simulink library "SUB_ECU_L4_MABX_HW_Interface"  (R2018a)
settings: Solver=VariableStepAuto  StartTime=0.0  StopTime=10.0  RelTol=1e-3
PostLoadFcn:
  | , if any(exist('dsrtsu_mdlpostloadfcn', 'file') == [2, 3, 6]), try dsrtsu_mdlpostloadfcn('Execute', bdroot); catch fprintf('Error in PostLoadFcn (dsrtsu_mdlpostloadfcn) for model "%s":\n %s\n', bdroot, lasterr); end, end,
undefined symbols (not defined in the file or in its folder): CANR_PROPB_REAX_3_13_CHANNEL_APV, CANR_PROPB_REAX_4_13_CHANNEL_APV, CANR_PROPB_XPR_1_50_CHANNEL_APV, ENUM_CAN_RX_T, ENUM_CAN_TX_T, ENUM_REAX_OPERATION_MODE_T, ENUM_SIGNAL_HEALTH_T, ENUM_XBR_CONTROL_MODE_T, ENUM_XBR_EBI_MODE_T, ENUM_XBR_PASS_THROUGH_ACTIVE_T, ENUM_XBR_PRIORITY_T, ENUM_XPR_INHIBIT_PARK_MANUAL_T, ENUM_XPR_INHIBIT_UNPARK_MANUAL_T, ENUM_XPR_PARK_MANUAL_T, ENUM_XPR_UNPARK_MANUAL_T, PROPB_REAX_1_E4_DES_POS_SIG_SRC_APV, PROPB_REAX_1_E4_DESIRED_OPMODE_APV, PROPB_REAX_1_E4_DESIRED_POSITION_APV, ptc_matlab_lib
libraries: PTC_MBDS_LIB x264, rtican x172, EmE_MBD_Blockset x39, simulink x34, $bdroot x16, rti1401lib_dio_type4 x8, simulink_need_slupdate x7, dsa_tcpip_lib x4, rti1401lib_adc_type4 x3, rtmapslib x3, rtitasklib x3
(part 9 of 51)

== system SUB_ECU_L4_MABX_HW_Interface/CAN_Out_PTC_1571/CAN_TX_10ms/Encode_PROPB_REAX_1 ==
  In1 : Inport
  Bus Selector : BusSelector  OutputSignals=10msTask.SteeringControl.DesSteeringAngle
  Bus Selector1 : BusSelector  OutputSignals=INPUTS.DIO_Bus.OperatorEnableSwitch
  CAN_ID_PropB_REAX_1_E4 : Subsystem
  Data Type Conversion : DataTypeConversion  OutDataTypeStr=uint8
  Encode_PROPB_REAX_1 : Subsystem
  PropB_REAX_1_E4_CommandFromExternalController : Subsystem
  PropB_REAX_1_E4_DesiredOperatingMode : Subsystem
  PropB_REAX_1_E4_MessageCounter : Subsystem
  Out1 : Outport
  wires:
  Data Type Conversion/1 -> PropB_REAX_1_E4_CommandFromExternalController/2(operatorEnable), PropB_REAX_1_E4_DesiredOperatingMode/1(OperatorEnable)
  Bus Selector/1 -> PropB_REAX_1_E4_CommandFromExternalController/1(DesiredSteeringAngle)  "<DesSteeringAngle>"
  Bus Selector1/1 -> Data Type Conversion/1  "<OperatorEnableSwitch>"
  CAN_ID_PropB_REAX_1_E4/1(MessageID) -> Encode_PROPB_REAX_1/1(MessageID)
  PropB_REAX_1_E4_DesiredOperatingMode/1(DesiredOperatingMode) -> Encode_PROPB_REAX_1/2(DesiredOperatingMode)
  Encode_PROPB_REAX_1/1(Data) -> Out1/1
  PropB_REAX_1_E4_MessageCounter/1(MessageCounter) -> Encode_PROPB_REAX_1/4(MessageCounter)
  PropB_REAX_1_E4_CommandFromExternalController/1(CommandFromExternalController) -> Encode_PROPB_REAX_1/3(CommandFromExternalController)
  In1/1 -> Bus Selector1/1, Bus Selector/1

== system SUB_ECU_L4_MABX_HW_Interface/CAN_Out_PTC_1571/CAN_TX_20ms/CAN_TX_PROPB_XBR_B3 ==
  Channel : Inport
  Data : Inport  Port=2
  OperatorEnable : Inport  Port=3
  AND : PTC_MBDS_LIB/MBDS Standard Library/Basic Operations/Logic and Bit Operations/AND  BitwiseMode=on  Inputs=1  UseBitMask=on  BitMask=bin2dec('00000001')  OutDataTypeStr=Inherit: Inherit via back propagation  PTC_MBDS_BlockVersion=5.41  PTC_BlockType=PTC_MBDS_AND
      settings: AttributesFormatString=bitwise  SourceProductName=PACCAR Technical Center MBDS Library
  Bus Selector2 : BusSelector  OutputSignals=XBRPassThroughActive
  Compare To Constant : simulink/Logic and Bit Operations/Compare To Constant  relop===  const=ENUM_XBR_PASS_THROUGH_ACTIVE_T.ACTIVE  OutDataTypeStr=boolean
  Data Type Conversion : DataTypeConversion  OutDataTypeStr=uint8  SaturateOnIntegerOverflow=on
  Data Type Conversion2 : DataTypeConversion  OutDataTypeStr=boolean  SaturateOnIntegerOverflow=on
  Logical Operator : Logic  AllPortsSameDT=off  OutDataTypeStr=boolean
  Logical Operator1 : Logic  Operator=OR  AllPortsSameDT=off  OutDataTypeStr=boolean
  Logical Operator7 : Logic  AllPortsSameDT=off  OutDataTypeStr=boolean
  Logical Operator8 : Logic  Operator=NOT  AllPortsSameDT=off  OutDataTypeStr=boolean
  TX_CAN1 : Subsystem
  Terminator : Terminator
  Unit_Delay : UnitDelay  InitialCondition=false  SampleTime=-1
      settings: AttributesFormatString=IC: %<vinit>
  wires:
  Compare To Constant/1 -> Terminator/1
  OperatorEnable/1 -> Unit_Delay/1, Logical Operator8/1, Logical Operator1/2
  Unit_Delay/1 -> Logical Operator7/1
  Logical Operator8/1 -> Logical Operator7/2
  Logical Operator/1 -> TX_CAN1/1(Enable)
  Logical Operator1/1 -> Logical Operator/1
  Logical Operator7/1 -> Logical Operator1/1
  Data Type Conversion2/1 -> Logical Operator/2
  Data/1 -> Bus Selector2/1, TX_CAN1/2(Data)
  Channel/1 -> Data Type Conversion/1
  Data Type Conversion/1 -> AND/1
  AND/1 -> Data Type Conversion2/1
  Bus Selector2/1 -> Compare To Constant/1  "<XBRPassThroughActive>"

== system SUB_ECU_L4_MABX_HW_Interface/CAN_Out_PTC_1571/CAN_TX_20ms/CAN_TX_STD_ODOMETRY ==
  Channel : Inport
  Data : Inport  Port=2
  AND : PTC_MBDS_LIB/MBDS Standard Library/Basic Operations/Logic and Bit Operations/AND  BitwiseMode=on  Inputs=1  UseBitMask=on  BitMask=bin2dec('00000001')  OutDataTypeStr=Inherit: Inherit via back propagation  PTC_MBDS_BlockVersion=5.41  PTC_BlockType=PTC_MBDS_AND
      settings: AttributesFormatString=bitwise  SourceProductName=PACCAR Technical Center MBDS Library
  AND1 : PTC_MBDS_LIB/MBDS Standard Library/Basic Operations/Logic and Bit Operations/AND  BitwiseMode=on  Inputs=1  UseBitMask=on  BitMask=bin2dec('00000010')  OutDataTypeStr=Inherit: Inherit via back propagation  PTC_MBDS_BlockVersion=5.41  PTC_BlockType=PTC_MBDS_AND
      settings: AttributesFormatString=bitwise  SourceProductName=PACCAR Technical Center MBDS Library
  AND2 : PTC_MBDS_LIB/MBDS Standard Library/Basic Operations/Logic and Bit Operations/AND  BitwiseMode=on  Inputs=1  UseBitMask=on  BitMask=bin2dec('00000100')  OutDataTypeStr=Inherit: Inherit via back propagation  PTC_MBDS_BlockVersion=5.41  PTC_BlockType=PTC_MBDS_AND
      settings: AttributesFormatString=bitwise  SourceProductName=PACCAR Technical Center MBDS Library
  AND3 : PTC_MBDS_LIB/MBDS Standard Library/Basic Operations/Logic and Bit Operations/AND  BitwiseMode=on  Inputs=1  UseBitMask=on  BitMask=bin2dec('00001000')  OutDataTypeStr=Inherit: Inherit via back propagation  PTC_MBDS_BlockVersion=5.41  PTC_BlockType=PTC_MBDS_AND
      settings: AttributesFormatString=bitwise  SourceProductName=PACCAR Technical Center MBDS Library
  AND4 : PTC_MBDS_LIB/MBDS Standard Library/Basic Operations/Logic and Bit Operations/AND  BitwiseMode=on  Inputs=1  UseBitMask=on  BitMask=bin2dec('00010000')  OutDataTypeStr=Inherit: Inherit via back propagation  PTC_MBDS_BlockVersion=5.41  PTC_BlockType=PTC_MBDS_AND
      settings: AttributesFormatString=bitwise  SourceProductName=PACCAR Technical Center MBDS Library
  AND5 : PTC_MBDS_LIB/MBDS Standard Library/Basic Operations/Logic and Bit Operations/AND  BitwiseMode=on  Inputs=1  UseBitMask=on  BitMask=bin2dec('00100000')  OutDataTypeStr=Inherit: Inherit via back propagation  PTC_MBDS_BlockVersion=5.41  PTC_BlockType=PTC_MBDS_AND
      settings: AttributesFormatString=bitwise  SourceProductName=PACCAR Technical Center MBDS Library
  Data Type Conversion : DataTypeConversion  OutDataTypeStr=uint8  SaturateOnIntegerOverflow=on
  Data Type Conversion{2..7} (6 alike) : DataTypeConversion  OutDataTypeStr=boolean  SaturateOnIntegerOverflow=on
  "Shift_Arithmetic " : ArithShift  BitShiftNumber=1
  Shift_Arithmetic 1 : ArithShift  BitShiftNumber=2
  Shift_Arithmetic 2 : ArithShift  BitShiftNumber=3
  Shift_Arithmetic 3 : ArithShift  BitShiftNumber=4
  Shift_Arithmetic 4 : ArithShift  BitShiftNumber=5
  TX_CAN6 : Subsystem
  Terminator{,1..9} (10 alike) : Terminator
  wires:
  Data Type Conversion7/1 -> TX_CAN6/1(Enable)
  Data Type Conversion6/1 -> Terminator5/1
  Data Type Conversion5/1 -> Terminator6/1
  Data Type Conversion4/1 -> Terminator7/1
  Data Type Conversion3/1 -> Terminator8/1
  Data Type Conversion2/1 -> Terminator9/1
  Data/1 -> Terminator4/1, Terminator3/1, Terminator2/1, Terminator1/1, Terminator/1, TX_CAN6/2(Data)
  AND1/1 -> "Shift_Arithmetic "/1
  AND2/1 -> Shift_Arithmetic 1/1
  Channel/1 -> Data Type Conversion/1
  Data Type Conversion/1 -> AND/1, AND1/1, AND4/1, AND5/1, AND3/1, AND2/1
  AND/1 -> Data Type Conversion2/1
  "Shift_Arithmetic "/1 -> Data Type Conversion3/1
  Shift_Arithmetic 1/1 -> Data Type Conversion4/1
  AND3/1 -> Shift_Arithmetic 2/1
  Shift_Arithmetic 2/1 -> Data Type Conversion5/1
  AND4/1 -> Shift_Arithmetic 3/1
  Shift_Arithmetic 3/1 -> Data Type Conversion6/1
  AND5/1 -> Shift_Arithmetic 4/1
  Shift_Arithmetic 4/1 -> Data Type Conversion7/1

== system SUB_ECU_L4_MABX_HW_Interface/CAN_Out_PTC_1571/CAN_TX_20ms/Encode_PropB_XBR_B3 ==
  note: This might cause a limit cycle, why switch pass through mode based on braking error
  In : Inport
  Bus Creator1 : BusCreator  Inputs=7
  Bus Creator2 : BusCreator  Inputs=7
  Bus Selector2 : BusSelector  OutputSignals=10msTask.BrakeCtrl.BrakingPID_Y,10msTask.BrakeCtrl.BrakingControlActive,INPUTS.DIO_Bus.OperatorEnableSwitch
  Constant10 : Constant  Value=ENUM_XBR_PASS_THROUGH_ACTIVE_T.NOT_ACTIVE
  Constant2 : Constant  Value=-15.687
  Constant4 : Constant  Value=0
  Constant7 : Constant  Value=ENUM_XBR_PASS_THROUGH_ACTIVE_T.ACTIVE
  Constant8 : Constant  Value=ENUM_XBR_PASS_THROUGH_ACTIVE_T.ERROR
  Constant9 : Constant  Value=ENUM_XBR_PASS_THROUGH_ACTIVE_T.NOT_AVAILABLE
  DECEL_GOV_XBR_URGENCY_MPV : Lookup_n-D  NumberOfTableDimensions=1  BreakpointsForDimension1=[-15.687 -2 -1.5 -1.2 -1.1 -1 -0.9 0]  Table=[100 50 20 15 15 15 10 10]  ExtrapMethod=Clip  UseLastTableValue=on  InputSameDT=on
      settings: AttributesFormatString=|
      | X: %<BreakpointsForDimension1>
      | Y: %<Table>
  Divide1 : Product  Inputs=**  InputSameDT=on
  If_Then_Else : EmE_MBD_Blockset/Signal Routing/If_Then_Else
      settings: SourceProductName=PACCAR EmE MBD Blockset
  Multiport Switch : MultiPortSwitch  DataPortOrder=Zero-based contiguous  Inputs=4  DiagnosticForDefault=None  zeroidx=on  InputSameDT=on
  Switch1 : Switch  Criteria=u2 ~= 0
  Terminator1 : Terminator
  XBRControlMode : Constant  Value=ENUM_XBR_CONTROL_MODE_T.ACCEL_CTRL_WITH_MAX_MODE
  XBRControlModeOVR : Constant  Value=ENUM_XBR_CONTROL_MODE_T.ACCEL_CTRL_WITH_MAX_MODE
  XBREnduranceBrakeIntegrationMode : Constant  Value=ENUM_XBR_EBI_MODE_T.EBI_ALLOWED
  XBREnduranceBrakeIntegrationModeOVR : Constant  Value=ENUM_XBR_EBI_MODE_T.EBI_ALLOWED
  XBRExternalAccelDemandOVR : Constant  Value=0
  XBRPassThroughActiveOVR : Constant  Value=ENUM_XBR_PASS_THROUGH_ACTIVE_T.ACTIVE
  XBRPassThroughEnabled : Constant
  XBRPassThroughEnabledOVR : Constant
  XBRPriority : Constant  Value=ENUM_XBR_PRIORITY_T.MEDIUM_PRIORITY
  XBRPriorityOVR : Constant  Value=ENUM_XBR_PRIORITY_T.MEDIUM_PRIORITY
  XBRUrgency : Constant  Value=25
  XBRUrgencyOVR : Constant  Value=25
  XBRValueOverride : Constant  Value=false
  Out : Outport
  wires:
  Constant4/1 -> Switch1/3
  Divide1/1 -> Switch1/1  "XBRExternalAccelDemand"
  Bus Selector2/3 -> Switch1/2  "<OperatorEnableSwitch>"
  Multiport Switch/1 -> Bus Creator1/5  "XBRPassThroughActive"
  DECEL_GOV_XBR_URGENCY_MPV/1 -> Terminator1/1  "XBRUrgency"
  Constant10/1 -> Multiport Switch/2
  Switch1/1 -> Bus Creator1/1, DECEL_GOV_XBR_URGENCY_MPV/1  "XBRExternalAccelDemand"
  Constant2/1 -> Divide1/2
  In/1 -> Bus Selector2/1
  Constant8/1 -> Multiport Switch/4
  Constant9/1 -> Multiport Switch/5
  Constant7/1 -> Multiport Switch/3
  XBREnduranceBrakeIntegrationMode/1 -> Bus Creator1/2  "XBREnduranceBrakeIntegrationMode"
  Bus Selector2/1 -> Divide1/1  "<BrakingPID_Y>"
  Bus Creator1/1 -> If_Then_Else/3
  XBRUrgency/1 -> Bus Creator1/6  "XBRUrgency"
  Bus Selector2/2 -> Multiport Switch/1  "<BrakingControlActive>"
  XBRControlMode/1 -> Bus Creator1/4  "XBRControlMode"
  XBRPriority/1 -> Bus Creator1/3  "XBRPriority"
  XBRPassThroughEnabled/1 -> Bus Creator1/7  "XBRPassThroughEnabled"
  XBRValueOverride/1 -> If_Then_Else/1
  If_Then_Else/1 -> Out/1
  XBRPassThroughActiveOVR/1 -> Bus Creator2/5  "XBRPassThroughActive"
  XBREnduranceBrakeIntegrationModeOVR/1 -> Bus Creator2/2  "XBREnduranceBrakeIntegrationMode"
  XBRExternalAccelDemandOVR/1 -> Bus Creator2/1  "XBRExternalAccelDemand"
  XBRUrgencyOVR/1 -> Bus Creator2/6  "XBRUrgency"
  XBRControlModeOVR/1 -> Bus Creator2/4  "XBRControlMode"
  XBRPriorityOVR/1 -> Bus Creator2/3  "XBRPriority"
  XBRPassThroughEnabledOVR/1 -> Bus Creator2/7  "XBRPassThroughEnabled"
  Bus Creator2/1 -> If_Then_Else/2

== system SUB_ECU_L4_MABX_HW_Interface/CAN_Out_PTC_1571/CAN_TX_5000ms/CAN_TX_RQST_13_E4 ==
  RawData : Inport
  OperatorEnable : Inport  Port=2
  Data Type Conversion6 : DataTypeConversion  OutDataTypeStr=boolean  SaturateOnIntegerOverflow=on
  Enable_TX_RequestDiagMsgFromREAX : Constant  Value=boolean(1)
  TX_CAN5 : Subsystem
  wires:
  OperatorEnable/1 -> TX_CAN5/3(OperatorEnable)
  Enable_TX_RequestDiagMsgFromREAX/1 -> Data Type Conversion6/1
  Data Type Conversion6/1 -> TX_CAN5/1(Enable)
  RawData/1 -> TX_CAN5/2(RawData)

== system SUB_ECU_L4_MABX_HW_Interface/CAN_Out_PTC_1571/CAN_TX_5000ms/Encode_RQST ==
  PGN : Inport
  AND : PTC_MBDS_LIB/MBDS Standard Library/Basic Operations/Logic and Bit Operations/AND  BitwiseMode=on  Inputs=1  UseBitMask=on  BitMask='000000FF'  OutDataTypeStr=uint8  PTC_MBDS_BlockVersion=5.41  PTC_BlockType=PTC_MBDS_AND
      settings: AttributesFormatString=bitwise  SourceProductName=PACCAR Technical Center MBDS Library
  AND1 : PTC_MBDS_LIB/MBDS Standard Library/Basic Operations/Logic and Bit Operations/AND  BitwiseMode=on  Inputs=1  UseBitMask=on  BitMask='0000FF00'  OutDataTypeStr=uint16  PTC_MBDS_BlockVersion=5.41  PTC_BlockType=PTC_MBDS_AND
      settings: AttributesFormatString=bitwise  SourceProductName=PACCAR Technical Center MBDS Library
  AND2 : PTC_MBDS_LIB/MBDS Standard Library/Basic Operations/Logic and Bit Operations/AND  BitwiseMode=on  Inputs=1  UseBitMask=on  BitMask='00FF0000'  OutDataTypeStr=uint32  PTC_MBDS_BlockVersion=5.41  PTC_BlockType=PTC_MBDS_AND
      settings: AttributesFormatString=bitwise  SourceProductName=PACCAR Technical Center MBDS Library
  Data Type Conversion : DataTypeConversion  OutDataTypeStr=uint32  SaturateOnIntegerOverflow=on
  Data Type Conversion1 : DataTypeConversion  OutDataTypeStr=uint8  SaturateOnIntegerOverflow=on
  Data Type Conversion2 : DataTypeConversion  OutDataTypeStr=uint8  SaturateOnIntegerOverflow=on
  Data Type Conversion3 : DataTypeConversion  OutDataTypeStr=uint8  SaturateOnIntegerOverflow=on
  Mux : Mux  Inputs=3
  "Shift_Arithmetic " : ArithShift  BitShiftNumber=8
  Shift_Arithmetic 1 : ArithShift  BitShiftNumber=16
  Data : Outport
  wires:
  Data Type Conversion3/1 -> Mux/1
  Mux/1 -> Data/1
  Data Type Conversion2/1 -> Mux/3
  Data Type Conversion1/1 -> Mux/2
  Shift_Arithmetic 1/1 -> Data Type Conversion2/1
  AND2/1 -> Shift_Arithmetic 1/1
  "Shift_Arithmetic "/1 -> Data Type Conversion1/1
  AND1/1 -> "Shift_Arithmetic "/1
  AND/1 -> Data Type Conversion3/1
  Data Type Conversion/1 -> AND/1, AND1/1, AND2/1
  PGN/1 -> Data Type Conversion/1

== system SUB_ECU_L4_MABX_HW_Interface/CAN_Out_PTC_1571/CAN_TX_5000ms/RQST_13_E4_PGN ==
  Repeating_Sequence_Stair : PTC_MBDS_LIB/Extras/Sources/Repeating_Sequence_Stair  OutValues=uint32([65527, 65226, 65227, 65235, 65242, 65259, 65267, 65260])  OutValues_prev=uint32([65527, 65226, 65227, 65235, 65242, 65259, 65267, 65260])  PTC_MBDS_BlockVersion=5.41  PTC_BlockType=PTC_MBDS_Repeating_Sequence_Stair
      settings: SourceProductName=PACCAR Technical Center MBDS Library
  PGN : Outport
  wires:
  Repeating_Sequence_Stair/1 -> PGN/1

== system SUB_ECU_L4_MABX_HW_Interface/CAN_Out_PTC_1571/CAN_TX_50ms/CAN_TX_CCVS1 ==
  In1 : Inport
  enable : Inport  Port=2
  Bus Selector : BusSelector  OutputSignals=INPUTS.CAN.CCVS1_00.CCVS1Data.TwoSpeedAxleSwitch,INPUTS.CAN.CCVS1_00.CCVS1Data.ParkingBrakeSwitch,INPUTS.CAN.CCVS1_00.CCVS1Data.CruiseCtrlPauseSwitch,INPUTS.CAN.CCVS1_00.CCVS1Data.ParkBrakeReleaseInhibitRq,INPUTS.CAN.CCVS1_00.CCVS1Data.WheelBasedVehicleSpeed,INPUTS.CAN.CCVS1_00.CCVS1Data.CruiseCtrlActive,INPUTS.CAN.CCVS1_00.CCVS1Data.CruiseCtrlEnableSwitch,INPUTS.CAN.CCVS1_00.CCVS1Data.BrakeSwitch,INPUTS.CAN.CCVS1_00.CCVS1Data.ClutchSwitch,INPUTS.CAN.CCVS1_00.CCVS1Data.CruiseCtrlSetSwitch,INPUTS.CAN.CCVS1_00.CCVS1Data.CruiseCtrlCoastSwitch,INPUTS.CAN.CCVS1_00.CCVS1Data.CruiseCtrlResumeSwitch,INPUTS.CAN.CCVS1_00.CCVS1Data.CruiseCtrlAccelerateSwitch,INPUTS.CAN.CCVS1_00.CCVS1Data.CruiseCtrlSetSpeed,INPUTS.CAN.CCVS1_00.CCVS1Data.PTOGovernorState,INPUTS.CAN.CCVS1_00.CCVS1Data.CruiseCtrlStates,INPUTS.CAN.CCVS1_00.CCVS1Data.EngIdleIncrementSwitch,INPUTS.CAN.CCVS1_00.CCVS1Data.EngIdleDecrementSwitch,INPUTS.CAN.CCVS1_00.CCVS1Data.EngTestModeSwitch,INPUTS.CAN.CCVS1_00.CCVS1Data.EngShutdownOverrideSwitch
  CCVS1_E3 : rtican/RTICAN Transmit (TX)   Reserved1=[]  Reserved2=[]  Reserved3=[]  Reserved4=[]  SfcnMessage=[]  Msg_Struct=[]  BoardTypeNo=[]  BoardNo=[]  ChannelNo=[]  Parameters=[]  DialogFcn=[]  UnitName=[]  Revision=[]  UnitValues=[]  DSProperties=struct('RTI',struct('Version',uint32(5),'BlockType',struct('isSLSource',uint8(1),'isSLSink',uint8(1),'isHWSource',uint8(0),'isHWSink',uint8(0),'isSetup',uint8(0),'isInline',uint8(1),'isNonInline',uint8(0),'isInterrupt',uint8(0),'isChannelwise',uint8(0)),'IOBoardType','RTICAN','UnitType','MESSAGE','Identifier','TX','DialogType','MSVC','BlockSet','RTICAN','SlaveProcessor','CAN'))  RTIBlockInterface=struct('InputPortsWidth',int32([1 1 1 1 1 1 1 1 1 1 1 1 1 1 1 1 1 1 1 1]),'InputPortsActive',ones(1,20),'InputPortsName',{{'SPN69_TwoSpeedAxleSwitch','SPN70_ParkingBrakeSwitch','SPN1633_CruiseControlPauseSwitch','SPN3807_ParkBrakeReleaseInhReq','SPN84_WheelBasedVehicleSpeed','SPN595_CruiseControlActive','SPN596_CruiseControlEnableSwitch','SPN597_BrakeSwitch','SPN598_ClutchSwitch','SPN599_CruiseControlSetSwitch','SPN600_CruiseControlCoastDecelSw','SPN601_CruiseControlResumeSwitch','SPN602_CruiseControlAccelerateSw','SPN86_CruiseControlSetSpeed','SPN976_PTOGovernorState','SPN527_CruiseControlStates','SPN968_EngIdleIncrementSw','SPN967_EngIdleDecrementSwitch','SPN966_EngDiagTestModeSwitch','SPN1237_EngShutdownOvrdSwitch'}},'InputPortsDataType',{{'SS_DOUBLE','SS_DOUBLE','SS_DOUBLE','SS_DOUBLE','SS_DOUBLE','SS_DOUBLE','SS_DOUBLE','SS_DOUBLE','SS_DOUBLE','SS_DOUBLE','SS_DOUBLE','SS_DOUBLE','SS_DOUBLE','SS_DOUBLE','SS_DOUBLE','SS_DOUBLE','SS_DOUBLE','SS_DOUBLE','SS_DOUBLE','SS_DOUBLE'}},'OutputPortsWidth',int32([1 1 1 1]),'OutputPortsActive',[1 1 1 1],'OutputPortsName',{{['TX status'],['TX time'],['TX delta time'],['TX delay time']}},'DialogFcn','rtican_message_interface_gui','BlockDisplay',{{'','center'}},'IconTransparency','on','InitLevel',3,'BlockName',struct('Token',{{'CCVS1_E3'}}),'SampleTime',{{-1}},'TriggerPort',{{'none'}},'EnablePort',{{'yes'}})  RTIBlockParameters="struct('BoardTypeNo',{{1,'OFF',[]}},'BoardNo',{{2,'ON',[1 16]}},'ChannelNo',{{1,'ON',[1 2]}},'Parameters',{{struct('DataFileSupport',struct('DataFileSelectedMaster',1,'DataFileSelectedLocal',1,'DataFileName','c:\\data\\svn\\truck1571\\dbc\\mabx_can1.dbc|','DataFileDate',{{{['10-Feb-2017 15:17:27']}}},'SelectedFile','dbc\\mabx_can1.dbc'),'Options',struct('StatusSelected',1,'TimeSelected',1,'DeltaTimeSelected',1,'DelayTimeSelected',1,'DelayTimeTXCommandSelected',0,'EncodeSetUnusedBitsToOne',0,'EnableMsgLoopback',0,'TriggerPort',struct('Selected',0,'TriggerType',0),'EnablePortSelected',1,'SignalOnPortnameSelected',1,'UserCoding',struct('Selected',0,'InterfaceFile','UserEncodingFile','FcnName','UserEncodeFcn','InportSelected',0,'InportWidth',1,'OutportSelected',0,'OutportWidth',1),'TerminationMsg',struct('Selected',0,'Byte0_7','0'),'InitialMsg',struct('Selected',0,'Byte0_7','0')),'Message',struct('MsgOnBlocknameSelected',1,'MsgName','CCVS1_E3','MsgIdFormat',1,'MsgId',419361251,'MsgLength',8,'NumSignals',20,'SampleTime',-1,'StartTime',struct('Selected',0,'Value',0),'AutoRepeatTime',struct('Selected',0,'Value',0.1),'Timeout',struct('Selected',0,'Value',0.1),'DelayTime',struct('Selected',0,'Value',0.1),'Signal',struct('SgnName',{'SPN69_TwoSpeedAxleSwitch','SPN70_ParkingBrakeSwitch','SPN1633_CruiseControlPauseSwitch','SPN3807_ParkBrakeReleaseInhReq','SPN84_WheelBasedVehicleSpeed','SPN595_CruiseControlActive','SPN596_CruiseControlEnableSwitch','SPN597_BrakeSwitch','SPN598_ClutchSwitch','SPN599_CruiseControlSetSwitch','SPN600_CruiseControlCoastDecelSw','SPN601_CruiseControlResumeSwitch','SPN602_CruiseControlAccelerateSw','SPN86_CruiseControlSetSpeed','SPN976_PTOGovernorState','SPN527_CruiseControlStates','SPN968_EngIdleIncrementSw','SPN967_EngIdleDecrementSwitch','SPN966_EngDiagTestModeSwitch','SPN1237_EngShutdownOvrdSwitch'},'SgnStartBit',{0,2,4,6,8,24,26,28,30,32,34,36,38,40,48,53,56,58,60,62},'SgnLength',{2,2,2,2,16,2,2,2,2,2,2,2,2,8,5,3,2,2,2,2},'SgnType',{0,0,0,0,0,0,0,0,0,0,0,0,0,0,0,0,0,0,0,0},'ModeValue',{-1,-1,-1,-1,-1,-1,-1,-1,-1,-1,-1,-1,-1,-1,-1,-1,-1,-1,-1,-1},'DataType',{0,0,0,0,0,0,0,0,0,0,0,0,0,0,0,0,0,0,0,0},'ByteLayout',{0,0,0,0,0,0,0,0,0,0,0,0,0,0,0,0,0,0,0,0},'Factor',{1,1,1,1,2^-8,1,1,1,1,1,1,1,1,1,1,1,1,1,1,1},'Offset',{0,0,0,0,0,0,0,0,0,0,0,0,0,0,0,0,0,0,0,0},'SgnComment',{{['Switch signal which indicates the current axle range.']},{['Switch signal which indicates when the parking brake is set.']},{['Switch signal which indicates the position of the Cruise Control Pause Switch used on Remote Cruise Control applications. The Cruise Control Pause Switch signal temporarily disables the Cruise Control function']},{['Park Brake Release Inhibit Request signals the desire that an applied park brake remain applied and limit the ability of the vehicle to be moved']},{['Speed of the vehicle as calculated from wheel or tailshaft speed.']},{['Cruise control is switched on or off']},{['Switch signal which indicates that it is possible to manage the cruise control function.']},{['Switch signal which indicates that the driver operated brake foot pedal is being pressed.']},{['Switch signal which indicates that the clutch pedal is being pressed.']},{['Switch signal of the cruise control activator which indicates that the activator is in the position “set.”']},{['Switch signal of the cruise control activator which indicates that the activator is in the position “coast (decelerate).”']},{['Switch signal of the cruise control activator which indicates that the activator is in the position “resume.”']},{['Switch signal of the cruise control activator which indicates that the activator is in the position “accelerate.”']},{['Value of set (chosen) velocity of velocity control system.  See SPN 6809 for an alternate resolution.']},{['This parameter is used to indicate the current state or mode of operation by the power takeoff (PTO) governor.']},{['This parameter is used to indicate the current state, or mode, of operation by the cruise control device.  This is a status parameter.']},{['Switch signal which indicates the position of the idle increment switch.']},{['Switch signal which indicates the position of the idle decrement switch.']},{['Switch signal which indicates the position of the engine diagnostic test mode switch.']},{['Switch signal which indicates the position of the engine shutdown override switch.  This switch function allows the operator to override an impending engine shutdown.']}},'SgnUnit',{'','','','','km/h','','','','','','','','','km/h','','','','','',''},'Min',{0,0,0,0,0,0,0,0,0,0,0,0,0,0,0,0,0,0,0,0},'Max',{0,0,0,0,0,0,0,0,0,0,0,0,0,0,0,0,0,0,0,0},'SLDataType',{'SS_DOUBLE','SS_DOUBLE','SS_DOUBLE','SS_DOUBLE','SS_DOUBLE','SS_DOUBLE','SS_DOUBLE','SS_DOUBLE','SS_DOUBLE','SS_DOUBLE','SS_DOUBLE','SS_DOUBLE','SS_DOUBLE','SS_DOUBLE','SS_DOUBLE','SS_DOUBLE','SS_DOUBLE','SS_DOUBLE','SS_DOUBLE','SS_DOUBLE'}),'MsgIdNumFormat',0,'MsgComment',{{['Cruise Control/Vehicle Speed 1 (Special CECU source address: 0xE3)']}}),'Version',1.2,'general',struct('isFromLib',0)),'OFF',[]}},'GroupId',{{struct('Group',{{'RTICAN'}},'No',3,'Behavior',{{'NAMECHANGE'}},'BlockType',{{'SINK'}},'NameChangeFlag',0),'OFF',[]}},'SFcnRTICANMessage',{{struct('MsgType','TX','SFcnPortType','Scalar','MsgName','CCVS1_E3','MsgIdFormat','XTD','MsgId',419361251,'MsgLength',8,'NumSignals',20,'SampleTime',-1,'StartTime',struct('Selected','no','Value',0),'AutoRepeatTime',struct('Selected','no','Value',0.1),'Timeout',struct('Selected','no','Value',0.1),'Signal',struct('SgnName',{'SPN69_TwoSpeedAxleSwitch','SPN70_ParkingBrakeSwitch','SPN1633_CruiseControlPauseSwitch','SPN3807_ParkBrakeReleaseInhReq','SPN84_WheelBasedVehicleSpeed','SPN595_CruiseControlActive','SPN596_CruiseControlEnableSwitch','SPN597_BrakeSwitch','SPN598_ClutchSwitch','SPN599_CruiseControlSetSwitch','SPN600_CruiseControlCoastDecelSw','SPN601_CruiseControlResumeSwitch','SPN602_CruiseControlAccelerateSw','SPN86_CruiseControlSetSpeed','SPN976_PTOGovernorState','SPN527_CruiseControlStates','SPN968_EngIdleIncrementSw','SPN967_EngIdleDecrementSwitch','SPN966_EngDiagTestModeSwitch','SPN1237_EngShutdownOvrdSwitch'},'SgnStartBit',{0,2,4,6,8,24,26,28,30,32,34,36,38,40,48,53,56,58,60,62},'SgnLength',{2,2,2,2,16,2,2,2,2,2,2,2,2,8,5,3,2,2,2,2},'SgnType',{'standard','standard','standard','standard','standard','standard','standard','standard','standard','standard','standard','standard','standard','standard','standard','standard','standard','standard','standard','standard'},'ModeValue',{-1,-1,-1,-1,-1,-1,-1,-1,-1,-1,-1,-1,-1,-1,-1,-1,-1,-1,-1,-1},'DataType',{['unsigned int'],['unsigned int'],['unsigned int'],['unsigned int'],['unsigned int'],['unsigned int'],['unsigned int'],['unsigned int'],['unsigned int'],['unsigned int'],['unsigned int'],['unsigned int'],['unsigned int'],['unsigned int'],['unsigned int'],['unsigned int'],['unsigned int'],['unsigned int'],['unsigned int'],['unsigned int']},'ByteLayout',{['little endian'],['little endian'],['little endian'],['little endian'],['little endian'],['little endian'],['little endian'],['little endian'],['little endian'],['little endian'],['little endian'],['little endian'],['little endian'],['little endian'],['little endian'],['little endian'],['little endian'],['little endian'],['little endian'],['little endian']},'Factor',{1,1,1,1,2^-8,1,1,1,1,1,1,1,1,1,1,1,1,1,1,1},'Offset',{0,0,0,0,0,0,0,0,0,0,0,0,0,0,0,0,0,0,0,0},'SLDataType',{'SS_DOUBLE','SS_DOUBLE','SS_DOUBLE','SS_DOUBLE','SS_DOUBLE','SS_DOUBLE','SS_DOUBLE','SS_DOUBLE','SS_DOUBLE','SS_DOUBLE','SS_DOUBLE','SS_DOUBLE','SS_DOUBLE','SS_DOUBLE','SS_DOUBLE','SS_DOUBLE','SS_DOUBLE','SS_DOUBLE','SS_DOUBLE','SS_DOUBLE'}),'StatusSelected','yes','TimeSelected','yes','DeltaTimeSelected','yes','DelayTimeSelected','yes','DelayTimeTXCommandSelected','no','EncodeSetUnusedBitsToOne','no','EnableMsgLoopback','no','TriggerPort',struct('Selected','no','TriggerType',0),'EnablePortSelected','yes','UserCoding',struct('Selected','no','InterfaceFile','UserEncodingFile','FcnName','UserEncodeFcn','InportSelected','no','InportWidth',1,'OutportSelected','no','OutportWidth',1),'TerminationMsg',struct('Selected','no','Byte0','0x00','Byte1','0x00','Byte2','0x00','Byte3','0x00','Byte4','0x00','Byte5','0x00','Byte6','0x00','Byte7','0x00'),'InitialMsg',struct('Selected','no','Byte0','0x00','Byte1','0x00','Byte2','0x00','Byte3','0x00','Byte4','0x00','Byte5','0x00','Byte6','0x00','Byte7','0x00'),'BoardType','DS1','BoardNo',2,'ControllerNo',1),'OFF',[]}},'TLCFileName',{{'rtican_tx_message','OFF',[]}})"  RTISFcnParameters=struct('SFcnRTICANMessage','struct','TLCFileName','char')  RTIBlockParaDefault=struct('BoardTypeNo',4302,'BoardNo',1,'ChannelNo',1,'Parameters',struct('DataFileSupport',struct('DataFileSelectedMaster',0,'DataFileSelectedLocal',0,'DataFileName','','DataFileDate','','SelectedFile',['<no file selected>']),'Options',struct('StatusSelected',1,'TimeSelected',1,'DeltaTimeSelected',1,'DelayTimeSelected',1,'DelayTimeTXCommandSelected',0,'EncodeSetUnusedBitsToOne',0,'EnableMsgLoopback',0,'TriggerPort',struct('Selected',0,'TriggerType','rising'),'EnablePortSelected',0,'SignalOnPortnameSelected',1,'UserCoding',struct('Selected',0,'InterfaceFile','UserEncodingFile','FcnName','UserEncodeFcn','InportSelected',0,'InportWidth',1,'OutportSelected',0,'OutportWidth',1),'TerminationMsg',struct('Selected',0,'Byte0_7','0'),'InitialMsg',struct('Selected',0,'Byte0_7','0')),'Message',struct('MsgOnBlocknameSelected',0,'MsgName',['TX Message'],'MsgIdFormat',0,'MsgId',100,'MsgLength',8,'NumSignals',1,'SampleTime',-1,'StartTime',struct('Selected',0,'Value',0),'AutoRepeatTime',struct('Selected',0,'Value',0.1),'Timeout',struct('Selected',0,'Value',0.1),'DelayTime',struct('Selected',0,'Value',0.1),'Signal',struct('SgnName',['TX signal'],'SgnStartBit',0,'SgnLength',8,'SgnType',0,'ModeValue',-1,'DataType',0,'SLDataType','SS_DOUBLE','ByteLayout',0,'Factor',1,'Offset',0,'Min',0,'Max',255,'SgnComment',{{}},'SgnUnit',''),'MsgIdNumFormat',0,'MsgComment',{{''}}),'Version',1.2,'general',struct('isFromLib',1)),'GroupId',struct('Group',{{'RTICAN'}},'No',1,'Behavior',{{'NAMECHANGE'}},'BlockType',{{'SINK'}},'NameChangeFlag',0),'SFcnRTICANMessage',struct('MsgType','TX','MsgName',['TX Message'],'MsgIdFormat','STD','MsgId',100,'MsgLength',2,'NumSignals',1,'SampleTime',-1,'StartTime',struct('Selected','no','Value',0),'AutoRepeatTime',struct('Selected','no','Value',0.1),'Timeout',struct('Selected','no','Value',0.1),'DelayTime',struct('Selected','no','Value',0.1),'Signal',struct('SgnName',['TX signal'],'SgnStartBit',0,'SgnLength',8,'SgnType','standard','ModeValue',-1,'DataType',['unsigned int'],'ByteLayout',['little endian'],'SLDataType','SS_DOUBLE','Factor',1,'Offset',0),'StatusSelected','yes','TimeSelected','yes','DeltaTimeSelected','yes','DelayTimeSelected','yes','EnablePortSelected','no','EnableMsgLoopback','no','DelayTimeTXCommandSelected','no','EncodeSetUnusedBitsToOne','no','UserCoding',struct('Selected','no','InterfaceFile','UserDecodingFile','FcnName','UserDecodeFcn','InportSelected','no','InportWidth',1,'OutportSelected','no','OutportWidth',1),'TerminationMsg',struct('Selected','no','Byte0','0x00','Byte1','0x00','Byte2','0x00','Byte3','0x00','Byte4','0x00','Byte5','0x00','Byte6','0x00','Byte7','0x00'),'InitialMsg',struct('Selected','no','Byte0','0x00','Byte1','0x00','Byte2','0x00','Byte3','0x00','Byte4','0x00','Byte5','0x00','Byte6','0x00','Byte7','0x00'),'TriggerPort',struct('Selected','no','TriggerType','rising'),'BoardType','DS4302','BoardNo',1,'ControllerNo',1,'SFcnPortType','Scalar'),'TLCFileName','rtican_tx_message')
      settings: AttributesFormatString=Group Id: RTICAN3\n  SourceProductName=dSPACE RTI CAN Blockset
  Terminator{,1..3} (4 alike) : Terminator
  wires:
  enable/1 -> CCVS1_E3/Enable
  Bus Selector/20 -> CCVS1_E3/20  "<EngShutdownOverrideSwitch>"
  Bus Selector/19 -> CCVS1_E3/19  "<EngTestModeSwitch>"
  Bus Selector/18 -> CCVS1_E3/18  "<EngIdleDecrementSwitch>"
  Bus Selector/17 -> CCVS1_E3/17  "<EngIdleIncrementSwitch>"
  Bus Selector/16 -> CCVS1_E3/16  "<CruiseCtrlStates>"
  Bus Selector/15 -> CCVS1_E3/15  "<PTOGovernorState>"
  Bus Selector/14 -> CCVS1_E3/14  "<CruiseCtrlSetSpeed>"
  Bus Selector/13 -> CCVS1_E3/13  "<CruiseCtrlAccelerateSwitch>"
  Bus Selector/12 -> CCVS1_E3/12  "<CruiseCtrlResumeSwitch>"
  Bus Selector/11 -> CCVS1_E3/11  "<CruiseCtrlCoastSwitch>"
  Bus Selector/10 -> CCVS1_E3/10  "<CruiseCtrlSetSwitch>"
  Bus Selector/9 -> CCVS1_E3/9  "<ClutchSwitch>"
  Bus Selector/8 -> CCVS1_E3/8  "<BrakeSwitch>"
  Bus Selector/7 -> CCVS1_E3/7  "<CruiseCtrlEnableSwitch>"
  Bus Selector/6 -> CCVS1_E3/6  "<CruiseCtrlActive>"
  Bus Selector/5 -> CCVS1_E3/5  "<WheelBasedVehicleSpeed>"
  Bus Selector/4 -> CCVS1_E3/4  "<ParkBrakeReleaseInhibitRq>"
  Bus Selector/3 -> CCVS1_E3/3  "<CruiseCtrlPauseSwitch>"
  Bus Selector/2 -> CCVS1_E3/2  "<ParkingBrakeSwitch>"
  Bus Selector/1 -> CCVS1_E3/1  "<TwoSpeedAxleSwitch>"
  CCVS1_E3/1 -> Terminator/1
  CCVS1_E3/2 -> Terminator1/1
  CCVS1_E3/3 -> Terminator2/1
  CCVS1_E3/4 -> Terminator3/1
  In1/1 -> Bus Selector/1
